simulink model "func_sim"  (R2014a)
settings: Solver=ode45  StartTime=0.0  StopTime=10.0  RelTol=1e-3
libraries: simulink x1
settings Model: Creator=BIgC46263347  LastModifiedBy=BIgC46263347

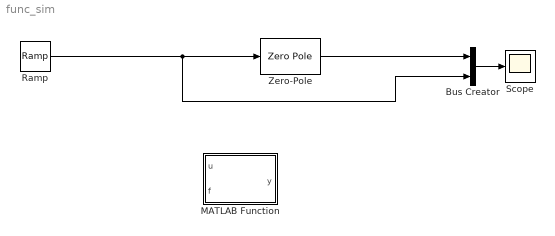
== system func_sim ==
  Bus Creator : BusCreator  Inputs=2
  MATLAB Function : MATLAB Function  TreatAsAtomicUnit=on
  Ramp : simulink/Sources/Ramp  slope=1  start=0  X0=0
  Scope : Scope
  Zero-Pole : ZeroPole  Zeros=[]  Poles=[-1/20]  Gain=[1/10]
  wires:
  Bus Creator/1 -> Scope/1
  Zero-Pole/1 -> Bus Creator/1
  Ramp/1 -> Bus Creator/2, Zero-Pole/1

== matlab function func_sim/MATLAB Function ==
  data: u input; y output; f input
function y = fcn(u,f)
gap=0.5
goal=3

if (f > goal+gap/2)
    y=0;
elseif (f < goal+gap/2)
    y=u;
end
